simulink model "drei_c"  (R2023a)
settings: Solver=VariableStepAuto  StartTime=0.0  StopTime=10.0  RelTol=1e-3
settings Model: Creator=alexa  LastModifiedBy=alexa

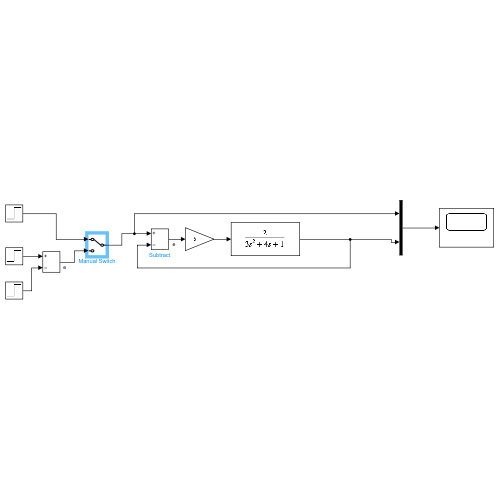
[thumbnail: Simulink's stored preview of the top-level diagram]
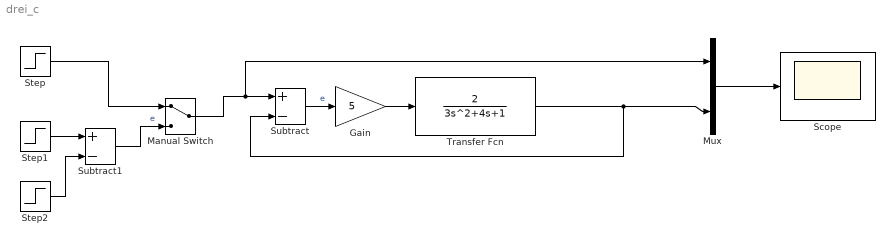
== system drei_c ==
  Gain : Gain  Gain=5
  Manual Switch : ManualSwitch
  Mux : Mux  Inputs=2
  Scope : Scope
  Step : Step  SampleTime=0
  Step1 : Step  After=10  SampleTime=0
  Step2 : Step  Time=1.1  After=10  SampleTime=0
  Subtract : Sum  Inputs=+-
  Subtract1 : Sum  Inputs=+-
  Transfer Fcn : TransferFcn  Numerator=[2]  Denominator=[3 4 1]
  wires:
  Subtract/1 -> Gain/1  "e"
  Gain/1 -> Transfer Fcn/1
  Transfer Fcn/1 -> Subtract/2, Mux/2
  Mux/1 -> Scope/1
  Step1/1 -> Subtract1/1
  Step2/1 -> Subtract1/2
  Subtract1/1 -> Manual Switch/2  "e"
  Step/1 -> Manual Switch/1
  Manual Switch/1 -> Mux/1, Subtract/1
